simulink model "car_kinetic"  (R2022a)
settings: Solver=FixedStepAuto  StartTime=0.0  StopTime=7  RelTol=1e-3
settings Model: Creator=yfx13  LastModifiedBy=yfx13

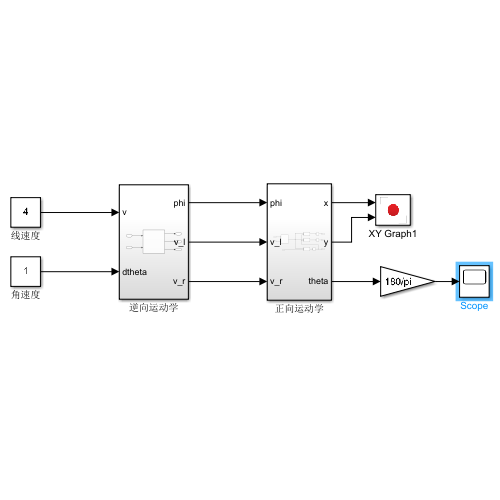
[thumbnail: Simulink's stored preview of the top-level diagram]
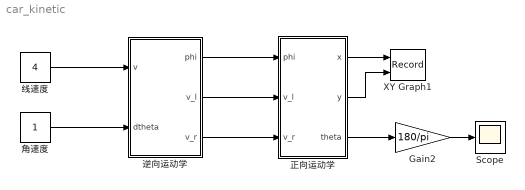
== system car_kinetic ==
  Gain2 : Gain  Gain=180/pi
  Scope : Scope
  XY Graph1 : Record  FileSettingsInternal="{\"entries\":[{\"content\":{\"excelSettings\":{\"content\":{},\"type\":\"Streamout.ExcelSettings\"}},\"type\":\"Streamout.FileSettingStorage\",\"uuid\":\"04fbfbed-5dd3-4ea5-8266-73876d63a9cb\"}],\"packageUris\":[\"http://schema.mathworks.com/mf0/streamout_blocks/R2020a\"],\"version\":\"1.0\"}"  Layout=[1 1]  SignalsInternal="{\"entries\":[{\"content\":{\"signals\":[{\"content\":{\"blockPath\":[\"car_like/XY Graph1\"],\"channel\":[],\"dimensions\":[1],\"domain\":\"car_like/XY Graph1\",\"lineColor\":\"#a2142f\",\"plots\":[1],\"port\":1,\"sid\":[\"\"],\"signalID\":3840,\"signalName\":\"正向运动学:1\"},\"type\":\"RecordBlkView.Signal\",\"uuid\":\"82e4e48a-2958-4a5e-9271-d9f6d61cdcc7\"},{\"content\":{\"blockPath\":[\"car_like/XY Graph1\"],\"channel\":[],\"dimensions\":[1],\"domain\":\"car_like/XY Graph1\",\"lineColor\":\"#139fff\",\"plots\":[1],\"port\":2,\"sid\":[\"\"],\"signalID\":3844,\"signalName\":\"正向运动学:2\"},\"type\":\"RecordBlkView.Signal\",\"uuid\":\"ea5d2f32-2d72-49a3-a222-36579f15b0ac\"}]},\"type\":\"RecordBlkView.InputSignals\",\"uuid\":\"20d9f353-b4be-4278-82cf-86b9d30eaa5a\"}],\"packageUris\":[\"http://schema.mathworks.com/mf0/streamout_blocks/R2020a\"],\"version\":\"1.0\"}"  VisualizationBindings="{\"xyplotplugin\":{\"info\":[{\"series\":[{\"bindingParametersList\":[{\"parameter\":\"X-Axis\",\"signalID\":3840,\"signalName\":\"正向运动学:1\"},{\"parameter\":\"Y-Axis\",\"signalID\":3844,\"signalName\":\"正向运动学:2\"}],\"seriesID\":31400}],\"subplotID\":1}]}}"  CompatibilityTag=XY
  正向运动学 : Subsystem
  线速度 : Constant  Value=4
  角速度 : Constant
  逆向运动学 : Subsystem
  wires:
  逆向运动学/1(phi) -> 正向运动学/1(phi)
  逆向运动学/2(v_l) -> 正向运动学/2(v_l)
  逆向运动学/3(v_r) -> 正向运动学/3(v_r)
  正向运动学/1(x) -> XY Graph1/1
  正向运动学/2(y) -> XY Graph1/2
  正向运动学/3(theta) -> Gain2/1
  Gain2/1 -> Scope/1
  角速度/1 -> 逆向运动学/2(dtheta)
  线速度/1 -> 逆向运动学/1(v)

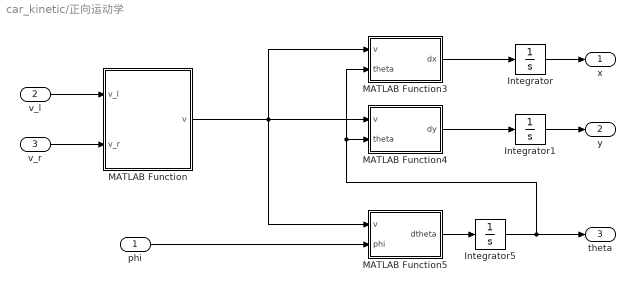
== system car_kinetic/正向运动学 ==
  phi : Inport
  v_l : Inport  Port=2
  v_r : Inport  Port=3
  Integrator : Integrator  InitialCondition=0.0001
  Integrator1 : Integrator
  Integrator5 : Integrator
  MATLAB Function : MATLAB Function  TreatAsAtomicUnit=on
  MATLAB Function3 : MATLAB Function  TreatAsAtomicUnit=on
  MATLAB Function4 : MATLAB Function  TreatAsAtomicUnit=on
  MATLAB Function5 : MATLAB Function  TreatAsAtomicUnit=on
  x : Outport
  y : Outport  Port=2
  theta : Outport  Port=3
  wires:
  MATLAB Function5/1(dtheta) -> Integrator5/1
  phi/1 -> MATLAB Function5/2(phi)
  MATLAB Function3/1(dx) -> Integrator/1
  Integrator/1 -> x/1
  Integrator1/1 -> y/1
  MATLAB Function4/1(dy) -> Integrator1/1
  Integrator5/1 -> MATLAB Function3/2(theta), MATLAB Function4/2(theta), theta/1
  MATLAB Function/1(v) -> MATLAB Function3/1(v), MATLAB Function5/1(v), MATLAB Function4/1(v)
  v_l/1 -> MATLAB Function/1(v_l)
  v_r/1 -> MATLAB Function/2(v_r)

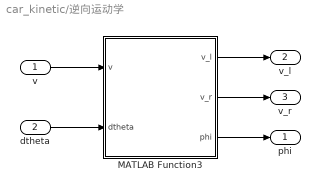
== system car_kinetic/逆向运动学 ==
  v : Inport
  dtheta : Inport  Port=2
  MATLAB Function3 : MATLAB Function  TreatAsAtomicUnit=on
  phi : Outport
  v_l : Outport  Port=2
  v_r : Outport  Port=3
  wires:
  dtheta/1 -> MATLAB Function3/2(dtheta)
  v/1 -> MATLAB Function3/1(v)
  MATLAB Function3/1(v_l) -> v_l/1
  MATLAB Function3/2(v_r) -> v_r/1
  MATLAB Function3/3(phi) -> phi/1

== matlab function car_kinetic/正向运动学/MATLAB Function3 ==
  data: v input; dx output; theta input
function dx = fcn(v,theta)
dx=v*cos(theta);

== matlab function car_kinetic/正向运动学/MATLAB Function4 ==
  data: v input; dy output; theta input
function dy = fcn(v,theta)
dy=v*sin(theta);

== matlab function car_kinetic/正向运动学/MATLAB Function5 ==
  data: v input; dtheta output; phi input
function dtheta = fcn(v,phi)
L=0.28;
dtheta=v*tan(phi)/L;

== matlab function car_kinetic/正向运动学/MATLAB Function ==
  data: v_l input; v output; v_r input
function v = fcn(v_l,v_r)
v=(v_l+v_r)/2;

== matlab function car_kinetic/逆向运动学/MATLAB Function3 ==
  data: v input; dtheta input; v_l output; v_r output; phi output
function [v_l,v_r,phi] = fcn(v,dtheta)
W=0.18;%宽度
L=0.28;
R=v/dtheta;   %L/phi;

v_l = (v/R)*(R-W/2);
v_r = (v/R)*(R+W/2);

phi_l=atan(L/(R-W/2));
phi_r=atan(L/(R+W/2));
phi=(phi_l+phi_r)/2;
if phi>pi/2
    phi=pi/2;
end
